simulink model "LaneTracking"  (R2023b)
settings: Solver=VariableStepAuto  StartTime=0.0  StopTime=Te  RelTol=1e-3
values from neighbouring files (symbols this model uses):
  Ts = 0.1    [ScriptBoot.m]    (also in ScriptBoot_TEST.m)
undefined symbols (not defined in the file or in its folder): driving, egoCarID, targetSpeed
libraries: drivingscenarioandsensors x7, robotcorelib x2, sensorinslib x1
(part 3 of 3)

== matlab function LaneTracking/Lane Boundaries to centerline/transform waypoints to world frame ==
  settings: sampleTime=Ts
  data: relativeWaypoints input; waypoints_worldframe output size=[300 2]; position input; yaw input
function waypoints_worldframe = transformWaypointsToWorld(relativeWaypoints, position, yaw)
    % Preallocate array for waypoints in world frame
    numPoints = size(relativeWaypoints, 1);
    waypoints_worldframe = zeros(numPoints, 2); % Assuming 2D waypoints [x, y]

    % Rotation matrix based on yaw angle
    R = [cos(yaw), -sin(yaw); sin(yaw), cos(yaw)];

    % Transform each waypoint
    for i = 1:numPoints
        % Rotate and translate waypoint
        waypoints_worldframe(i, :) = (R * relativeWaypoints(i, :)')' + position';
    end
end

== matlab function LaneTracking/Lane Boundaries to centerline/calculate lane centerline  ==
  settings: sampleTime=Ts
  data: curvatureLeft input; centerlineWaypoints output size=[300, 2]; curvelengthLeft input; headingangleLeft input; lateraloffsetLeft input; curvatureRight input; curvelengthRight input; headingangleRight input; lateraloffsetRight input; targetCruiseSpeed input
function centerlineWaypoints = calculateLaneCenterline(curvatureLeft, curvelengthLeft, headingangleLeft, lateraloffsetLeft, curvatureRight, curvelengthRight, headingangleRight, lateraloffsetRight, targetCruiseSpeed)
    % Calculate the average curvature, curve length, heading angle, and lateral offset
    curvature = (curvatureLeft + curvatureRight) / 2;
    curvelength = (curvelengthLeft + curvelengthRight) / 2;
    headingangle = (headingangleLeft + headingangleRight) / 2;
    lateraloffset = (lateraloffsetLeft + lateraloffsetRight) / 2;

    % Estimate the optimal number of waypoints
    updateInterval = 0.1; % seconds
    distancePerUpdate = targetCruiseSpeed * updateInterval;
    totalDistance = sum(curvelength,'all');
    numPoints = max(10, ceil(totalDistance / distancePerUpdate)); % Ensure at least 10 points for very short curves

    % Preallocate array for waypoints
    % centerlineWaypoints = zeros(numPoints, 2); % [x, y] format
    centerlineWaypoints = NaN(300, 2); % [x, y] format

    % Generate waypoints along the centerline
    for i = 1:numPoints
        t = (i - 1) / (numPoints - 1); % Normalized distance along the lane

        % Calculate x and y coordinates of the centerline waypoints
        x = curvelength * t * cosd(headingangle);
        y = curvelength * t * sind(headingangle) + lateraloffset;

        centerlineWaypoints(i, :) = [x, y];
    end
end

== matlab function LaneTracking/Environment/Pack Ego Actor ==
  data: pos input; a output Bus: BusActorsActors size=1; vel input; yaw input; yawRate input; ActorID input
function a = packEgo(pos,vel,yaw,yawRate,ActorID)
% Pack ego information into a single ego actor bus
%
% Imoprtant note:
% Output is a bus of type BusActorsActors. This is the same bus used by the
% Scenario Reader to output an individual actor. If you change the
% output bus name of Scenario Reader change the output bus name here
% as well by clicking on 'Edit Data' in the menu above.

a = struct(...
    'ActorID',ActorID,...
    'Position', [pos(1) pos(2) 0], ...
    'Velocity', [vel(1) vel(2) 0], ...
    'Roll', 0, ...
    'Pitch', 0, ...
    'Yaw', yaw, ...
    'AngularVelocity', [0 0 yawRate]);
